simulink model "Decryption_App"  (R2023a)
settings: Solver=FixedStepAuto  StartTime=0.0  StopTime=10.0  RelTol=1e-3
libraries: androiduilib x3, dspsrcs4 x2, androidaudiovideolib x1, androidcommunicationlib x1
settings Model: Creator=ragha  LastModifiedBy=ragha
settings OptimizationCC: EnhancedBackFolding=on  PassReuseOutputArgsAs=Individual arguments  ZeroExternalMemoryAtStartup=off  ZeroInternalMemoryAtStartup=off  MaxStackSize=64  OptimizeBlockOrder=speed  DifferentSizesBufferReuse=on  OptimizationCustomize=off  EfficientTunableParamExpr=on
settings DebuggingCC: ParameterTunabilityLossMsg=error
settings HardwareCC: ProdBitPerPointer=32  ProdBitPerSizeT=32  ProdBitPerPtrDiffT=32  ProdLargestAtomicInteger=Long  ProdLargestAtomicFloat=Double  ProdWordSize=32  ProdHWDeviceType=ARM Compatible->ARM Cortex
settings SFSimCC: MATLABDynamicMemAlloc=off
settings RTWCC: Description=Embedded Coder  SystemTargetFile=ert.tlc  HardwareBoard=Android Device  TLCOptions="-aInlineSetEventsForThisBaseRateFcn=TLC_FALSE -aSuppressMultiTaskScheduler=TLC_FALSE  -aRateBasedStepFcn=0"  TemplateMakefile=ert_default_tmf  RTWVerbose=off  Toolchain=Android SDK/NDK Tools
settings CodeAppCC: ForceParamTrailComments=on  IgnoreCustomStorageClasses=off  OperatorAnnotations=on  SimulinkDataObjDesc=on  SFDataObjDesc=on  InsertBlockDesc=on

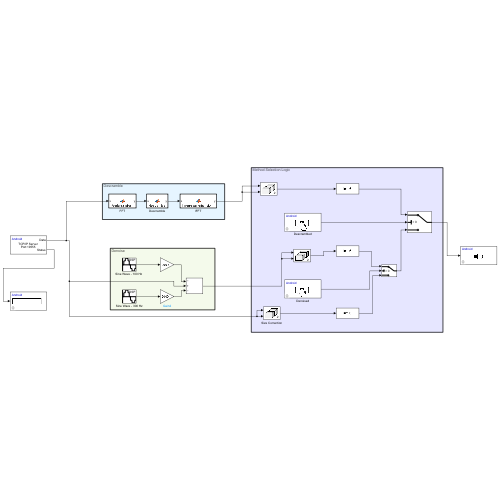
[thumbnail: Simulink's stored preview of the top-level diagram]
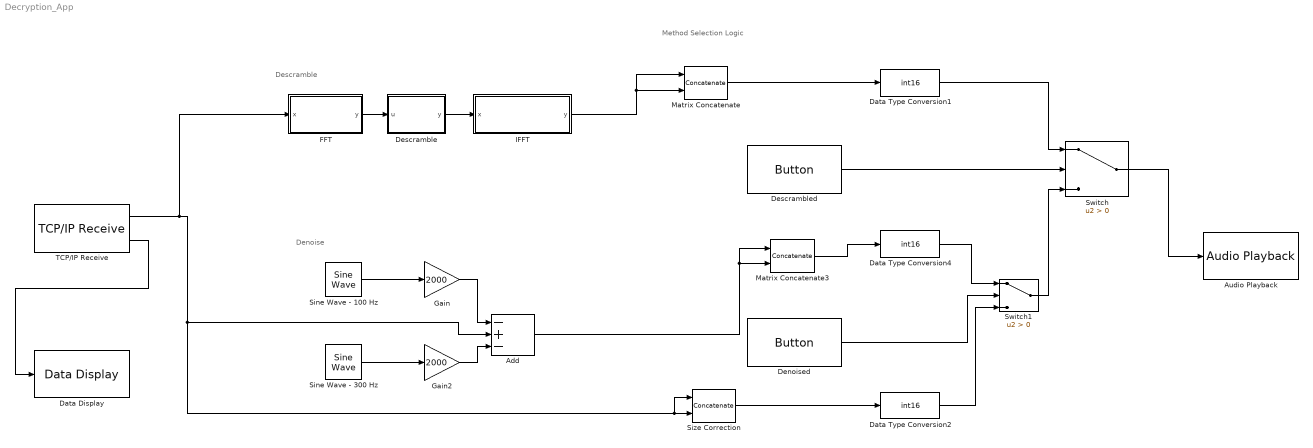
== system Decryption_App ==
  note: Method Selection Logic
  note: Descramble
  note: Denoise
  Add : Sum  Inputs=-+-
  Audio Playback : androidaudiovideolib/Audio Playback  SampleFreq=44100  AudioSamplingFreq=44100  SampleTime=0.1  DeviceStr=0  QueueDuration=0  BlockPlatform=Android
  Data Display : androiduilib/Data Display  DataDisplayId=Decryption_App/Data_Display  Format=Float  Precision=6  SimulateUsing=Code generation  blockPlatform=Android
  Data Type Conversion1 : DataTypeConversion  OutDataTypeStr=int16  RndMeth=Nearest  SaturateOnIntegerOverflow=off
  Data Type Conversion2 : DataTypeConversion  OutDataTypeStr=int16  RndMeth=Nearest  SaturateOnIntegerOverflow=off
  Data Type Conversion4 : DataTypeConversion  OutDataTypeStr=int16  RndMeth=Nearest  SaturateOnIntegerOverflow=off
  Denoised : androiduilib/Button  ButtonState=Not pressed  ButtonId=Decryption_App/Denoised  State=off  SampleTime=0.1  BlockPlatform=Android
  Descramble : MATLAB Function  TreatAsAtomicUnit=on
  "Descrambled " : androiduilib/Button  ButtonState=Not pressed  ButtonId=Decryption_App/Descrambled_  State=off  SampleTime=0.1  BlockPlatform=Android
  FFT : MATLAB Function  TreatAsAtomicUnit=on
  Gain : Gain  Gain=2000
  Gain2 : Gain  Gain=2000
  IFFT : MATLAB Function  TreatAsAtomicUnit=on
  Matrix Concatenate : Concatenate  Mode=Multidimensional array  ConcatenateDimension=2
  Matrix Concatenate3 : Concatenate  Mode=Multidimensional array  ConcatenateDimension=2
  "Sine Wave - 100 Hz " : dspsrcs4/Sine Wave  Amplitude=1  Frequency=100  Phase=0  SampleMode=Discrete  OutComplex=Real  CompMethod=Trigonometric fcn  TableSize=Speed  SampleTime=1/1000  SamplesPerFrame=1  ResetState=Restart at time zero  OutputFrames=off  dataType=double  wordLen=16  udDataType=sfix(16)  fracBitsMode=Best precision  numFracBits=15  OutDataTypeStr=double  LastOutDataTypeStr=double
  Sine Wave - 300 Hz : dspsrcs4/Sine Wave  Amplitude=1  Frequency=300  Phase=0  SampleMode=Discrete  OutComplex=Real  CompMethod=Trigonometric fcn  TableSize=Speed  SampleTime=1/1000  SamplesPerFrame=1  ResetState=Restart at time zero  OutputFrames=off  dataType=double  wordLen=16  udDataType=sfix(16)  fracBitsMode=Best precision  numFracBits=15  OutDataTypeStr=double  LastOutDataTypeStr=double
  Size Correction : Concatenate  Mode=Multidimensional array  ConcatenateDimension=2
  Switch : Switch  Criteria=u2 > Threshold  SaturateOnIntegerOverflow=off  InputSameDT=off
  Switch1 : Switch  Criteria=u2 > Threshold  SaturateOnIntegerOverflow=off  InputSameDT=off
  TCP/IP Receive : androidcommunicationlib/TCP//IP Receive  TCPReceiveId=Decryption_App/TCP//IP_Receive  Mode_=Server  LocalServerPort_=19555  RemoteAddr_=127.0.0.1  RemoteServerPort_=25000  DataType_=double  DataSize_=441  SampleTime_=0.01  ClientPortBindingSelection_=off  ClientPortToBind_=35000  BlockingMode_=off  BlockTimeout_=0.1
  wires:
  Matrix Concatenate/1 -> Data Type Conversion1/1
  TCP/IP Receive/2 -> Data Display/1
  Descramble/1(y) -> IFFT/1(x)
  FFT/1(y) -> Descramble/1(u)
  IFFT/1(y) -> Matrix Concatenate/1, Matrix Concatenate/2
  Switch/1 -> Audio Playback/1
  Data Type Conversion1/1 -> Switch/1
  "Descrambled "/1 -> Switch/2
  TCP/IP Receive/1 -> FFT/1(x), Add/2, Size Correction/1, Size Correction/2
  Size Correction/1 -> Data Type Conversion2/1
  Denoised/1 -> Switch1/2
  Switch1/1 -> Switch/3
  Data Type Conversion2/1 -> Switch1/3
  Matrix Concatenate3/1 -> Data Type Conversion4/1
  Data Type Conversion4/1 -> Switch1/1
  Sine Wave - 300 Hz/1 -> Gain2/1
  Add/1 -> Matrix Concatenate3/1, Matrix Concatenate3/2
  "Sine Wave - 100 Hz "/1 -> Gain/1
  Gain2/1 -> Add/3
  Gain/1 -> Add/1

== matlab function Decryption_App/IFFT ==
  data: x input; y output
function y = inversefouriertransform(x)
    y = real(ifft(x));
end

== matlab function Decryption_App/Descramble ==
  data: u input; y output
function y = descramble(u)

y = u/6;

== matlab function Decryption_App/FFT ==
  data: x input; y output
function y = fouriertransform(x)
    y = fft(x);
end
